simulink model "test07_bis"  (Simulink 7.4)
settings: Solver=ode3  StartTime=0.0  StopTime=inf  RelTol=1e-3
undefined symbols (not defined in the file or in its folder): serial
libraries: NAV420Lib x4, instrumentlib x3
settings Model: Creator=djulzz  LastModifiedBy=djulzz
settings DebuggingCC: SolverPrmCheckMsg=none

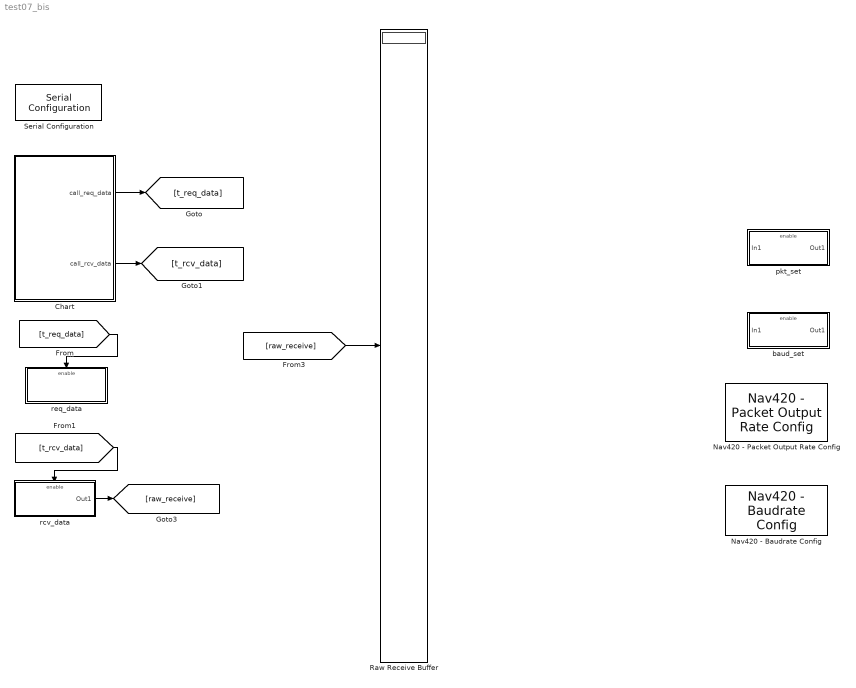
== system test07_bis ==
  Chart : Stateflow chart
  Nav420 - Baudrate Config : NAV420Lib/Nav420 - Baudrate Config  SystemSampleTime=-1  baudrateIndex=9600  SaveConfig=off
  Nav420 - Packet Output Rate Config : NAV420Lib/Nav420 - Packet Output Rate Config  SystemSampleTime=-1  shouldSave=off  output_rate=100
  Raw Receive Buffer : Display
      settings: Format=hex (Stored Integer)
  Serial Configuration : instrumentlib/Serial Configuration  Priority=-200000  DialogController=instrumentcreatedialog  DialogControllerArgs=DataTag0  ComPortMenu=COM1  ComPort=COM1  ObjConstructor=serial('COM1');  BaudRate=38400  DataBits=8  Parity=none  StopBits=1  FlowControl=none  Timeout=10  ByteOrder=LittleEndian
  baud_set : Subsystem  TreatAsAtomicUnit=on
  pkt_set : Subsystem  TreatAsAtomicUnit=on
  rcv_data : Subsystem  TreatAsAtomicUnit=on
  req_data : Subsystem  TreatAsAtomicUnit=on
  wires:
  Chart/1(call_req_data) -> [t_req_data]
  Chart/2(call_rcv_data) -> [t_rcv_data]
  [raw_receive] -> Raw Receive Buffer/1
  rcv_data/1(Out1) -> [raw_receive]
  [t_req_data] -> req_data/Enable
  [t_rcv_data] -> rcv_data/Enable

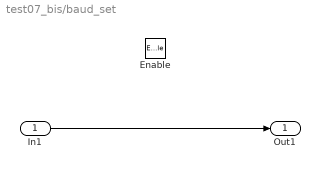
== system test07_bis/baud_set ==
  In1 : Inport  OutDataType=fixdt(1, 16)  OutScaling=2^0
  Enable : EnablePort
  Out1 : Outport  OutDataType=fixdt(1, 16)  OutScaling=2^0
  wires:
  In1/1 -> Out1/1

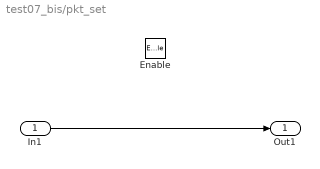
== system test07_bis/pkt_set ==
  In1 : Inport  OutDataType=fixdt(1, 16)  OutScaling=2^0
  Enable : EnablePort
  Out1 : Outport  OutDataType=fixdt(1, 16)  OutScaling=2^0
  wires:
  In1/1 -> Out1/1

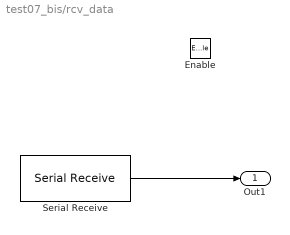
== system test07_bis/rcv_data ==
  Enable : EnablePort
  Serial Receive : instrumentlib/Serial Receive  DialogController=instrumentcreatedialog  DialogControllerArgs=DataTag1  ComPortMenu=COM1  ComPort=COM1  ObjConstructor=serial('COM1');  Terminator=<none>  DataSize="[35   1]"  DataType=uint8  EnableBlockingMode=on  ActionDataUnavailable=Output last received value  CustomValue=0  SampleTime=-1
  Out1 : Outport  DataType=uint8  OutDataType=fixdt(1, 16)  OutScaling=2^0  OutDataTypeStr=uint8
  wires:
  Serial Receive/1 -> Out1/1

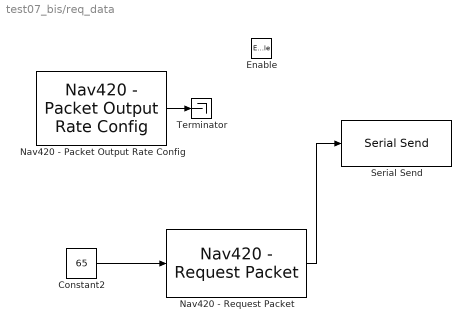
== system test07_bis/req_data ==
  Enable : EnablePort
  Constant2 : Constant  Value=65  OutDataTypeMode=int8  OutDataType=fixdt(1, 16)  OutScaling=2^0  OutDataTypeStr=int8  SampleTime=-1
  Nav420 - Packet Output Rate Config : NAV420Lib/Nav420 - Packet Output Rate Config  SystemSampleTime=-1  shouldSave=on  output_rate=0
  Nav420 - Request Packet : NAV420Lib/Nav420 - Request Packet  SystemSampleTime=-1
  Serial Send : instrumentlib/Serial Send  DialogController=instrumentcreatedialog  DialogControllerArgs=DataTag2  ComPortMenu=COM1  ComPort=COM1  ObjConstructor=serial('COM1');  Terminator=<none>  EnableBlockingMode=on
  Terminator : Terminator
  wires:
  Constant2/1 -> Nav420 - Request Packet/1
  Nav420 - Packet Output Rate Config/1 -> Terminator/1
  Nav420 - Request Packet/1 -> Serial Send/1

== stateflow chart Chart ==
  state Step1
    call_req_data=1;
  state Step2
    call_req_data=0;
  state Step3
    call_rcv_data=1;
  state Step4
    call_rcv_data=0;
  (default) -> Step1
  Step1 -> Step2
  Step2 -> Step3
  Step3 -> Step4
  Step4 -> Step1
  data: call_req_data output uint8; call_rcv_data output uint8
